simulink model "FCSSystem"  (R2025b)
settings: Solver=VariableStepAuto  StartTime=0.0  StopTime=10.0  RelTol=1e-3
settings Model: DataDictionary=FCSInterfaces.sldd  Creator=sarah  LastModifiedBy=sarah

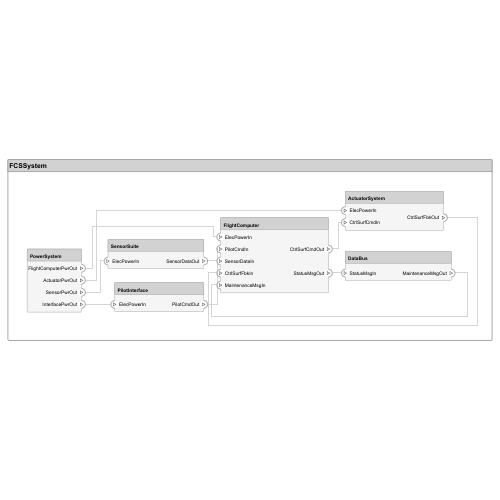
[thumbnail: Simulink's stored preview of the top-level diagram]
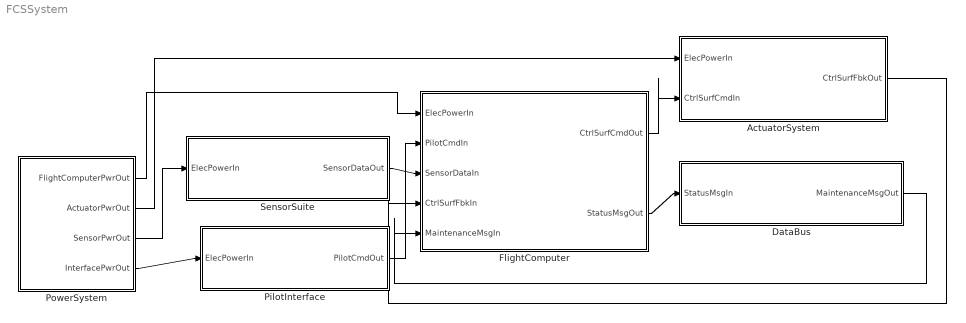
== system FCSSystem ==
  ActuatorSystem : Subsystem
      settings: PortSchema="{\"entries\":[{\"content\":{\"headerSize\":26,\"margin\":15,\"minimumSpacing\":25,\"sides\":[{\"content\":{\"connectorIds\":[\"In1\",\"In2\"]},\"type\":\"ConnectorPlacement.EquallySpacedRectSide\",\"uuid\":\"20d6bed0-d8e5-4088-8794-9345a2942e90\"},{\"content\":{\"connectorIds\":[\"Out1\"],\"side\":\"RIGHT\"},\"type\":\"ConnectorPlacement.EquallySpacedRectSide\",\"uuid\":\"e7adde65-1579-42e2-b600-0f533305a23b\"},{\"content\":{\"side\":\"TOP\"},\"type\":\"ConnectorPlacement.EquallySpacedRectSide\",\"uuid\":\"73636ec6-6908-4b74-b302-6e84b019a70e\"}]},\"type\":\"ConnectorPlacement.EquallySpacedConnector\",\"uuid\":\"cc5d9ea4-0f09-4026-9dcf-92b706ac45bf\"}],\"packageUris\":[\"http://schema.mathworks.com/mf0/Connector/R2020b\"],\"version\":\"1.0\"}"
  DataBus : Subsystem
      settings: PortSchema="{\"entries\":[{\"content\":{\"headerSize\":26,\"margin\":15,\"minimumSpacing\":25,\"sides\":[{\"content\":{\"connectorIds\":[\"In1\"]},\"type\":\"ConnectorPlacement.EquallySpacedRectSide\",\"uuid\":\"20d6bed0-d8e5-4088-8794-9345a2942e90\"},{\"content\":{\"connectorIds\":[\"Out1\"],\"side\":\"RIGHT\"},\"type\":\"ConnectorPlacement.EquallySpacedRectSide\",\"uuid\":\"e7adde65-1579-42e2-b600-0f533305a23b\"},{\"content\":{\"side\":\"TOP\"},\"type\":\"ConnectorPlacement.EquallySpacedRectSide\",\"uuid\":\"73636ec6-6908-4b74-b302-6e84b019a70e\"}]},\"type\":\"ConnectorPlacement.EquallySpacedConnector\",\"uuid\":\"cc5d9ea4-0f09-4026-9dcf-92b706ac45bf\"}],\"packageUris\":[\"http://schema.mathworks.com/mf0/Connector/R2020b\"],\"version\":\"1.0\"}"
  FlightComputer : Subsystem
      settings: PortSchema="{\"entries\":[{\"content\":{\"headerSize\":26,\"margin\":15,\"minimumSpacing\":25,\"sides\":[{\"content\":{\"connectorIds\":[\"In1\",\"In2\",\"In3\",\"In4\",\"In5\"]},\"type\":\"ConnectorPlacement.EquallySpacedRectSide\",\"uuid\":\"20d6bed0-d8e5-4088-8794-9345a2942e90\"},{\"content\":{\"connectorIds\":[\"Out1\",\"Out2\"],\"side\":\"RIGHT\"},\"type\":\"ConnectorPlacement.EquallySpacedRectSide\",\"uuid\":\"e7adde65-1579-42e2-b600-0f533305a23b\"},{\"content\":{\"side\":\"TOP\"},\"type\":\"ConnectorPlacement.EquallySpacedRectSide\",\"uuid\":\"73636ec6-6908-4b74-b302-6e84b019a70e\"}]},\"type\":\"ConnectorPlacement.EquallySpacedConnector\",\"uuid\":\"cc5d9ea4-0f09-4026-9dcf-92b706ac45bf\"}],\"packageUris\":[\"http://schema.mathworks.com/mf0/Connector/R2020b\"],\"version\":\"1.0\"}"
  PilotInterface : Subsystem
      settings: PortSchema="{\"entries\":[{\"content\":{\"headerSize\":26,\"margin\":15,\"minimumSpacing\":25,\"sides\":[{\"content\":{\"connectorIds\":[\"In1\"]},\"type\":\"ConnectorPlacement.EquallySpacedRectSide\",\"uuid\":\"20d6bed0-d8e5-4088-8794-9345a2942e90\"},{\"content\":{\"connectorIds\":[\"Out1\"],\"side\":\"RIGHT\"},\"type\":\"ConnectorPlacement.EquallySpacedRectSide\",\"uuid\":\"e7adde65-1579-42e2-b600-0f533305a23b\"},{\"content\":{\"side\":\"TOP\"},\"type\":\"ConnectorPlacement.EquallySpacedRectSide\",\"uuid\":\"73636ec6-6908-4b74-b302-6e84b019a70e\"}]},\"type\":\"ConnectorPlacement.EquallySpacedConnector\",\"uuid\":\"cc5d9ea4-0f09-4026-9dcf-92b706ac45bf\"}],\"packageUris\":[\"http://schema.mathworks.com/mf0/Connector/R2020b\"],\"version\":\"1.0\"}"
  PowerSystem : Subsystem
      settings: PortSchema="{\"entries\":[{\"content\":{\"headerSize\":26,\"margin\":15,\"minimumSpacing\":25,\"sides\":[{\"content\":{},\"type\":\"ConnectorPlacement.EquallySpacedRectSide\",\"uuid\":\"20d6bed0-d8e5-4088-8794-9345a2942e90\"},{\"content\":{\"connectorIds\":[\"Out1\",\"Out2\",\"Out3\",\"Out4\"],\"side\":\"RIGHT\"},\"type\":\"ConnectorPlacement.EquallySpacedRectSide\",\"uuid\":\"e7adde65-1579-42e2-b600-0f533305a23b\"},{\"content\":{\"side\":\"TOP\"},\"type\":\"ConnectorPlacement.EquallySpacedRectSide\",\"uuid\":\"73636ec6-6908-4b74-b302-6e84b019a70e\"}]},\"type\":\"ConnectorPlacement.EquallySpacedConnector\",\"uuid\":\"cc5d9ea4-0f09-4026-9dcf-92b706ac45bf\"}],\"packageUris\":[\"http://schema.mathworks.com/mf0/Connector/R2020b\"],\"version\":\"1.0\"}"
  SensorSuite : Subsystem
      settings: PortSchema="{\"entries\":[{\"content\":{\"headerSize\":26,\"margin\":15,\"minimumSpacing\":25,\"sides\":[{\"content\":{\"connectorIds\":[\"In1\"]},\"type\":\"ConnectorPlacement.EquallySpacedRectSide\",\"uuid\":\"20d6bed0-d8e5-4088-8794-9345a2942e90\"},{\"content\":{\"connectorIds\":[\"Out1\"],\"side\":\"RIGHT\"},\"type\":\"ConnectorPlacement.EquallySpacedRectSide\",\"uuid\":\"e7adde65-1579-42e2-b600-0f533305a23b\"},{\"content\":{\"side\":\"TOP\"},\"type\":\"ConnectorPlacement.EquallySpacedRectSide\",\"uuid\":\"73636ec6-6908-4b74-b302-6e84b019a70e\"}]},\"type\":\"ConnectorPlacement.EquallySpacedConnector\",\"uuid\":\"cc5d9ea4-0f09-4026-9dcf-92b706ac45bf\"}],\"packageUris\":[\"http://schema.mathworks.com/mf0/Connector/R2020b\"],\"version\":\"1.0\"}"
  wires:
  PowerSystem/4(InterfacePwrOut) -> PilotInterface/1(ElecPowerIn)
  PowerSystem/3(SensorPwrOut) -> SensorSuite/1(ElecPowerIn)
  DataBus/1(MaintenanceMsgOut) -> FlightComputer/5(MaintenanceMsgIn)
  PowerSystem/2(ActuatorPwrOut) -> ActuatorSystem/1(ElecPowerIn)
  PowerSystem/1(FlightComputerPwrOut) -> FlightComputer/1(ElecPowerIn)
  SensorSuite/1(SensorDataOut) -> FlightComputer/3(SensorDataIn)
  PilotInterface/1(PilotCmdOut) -> FlightComputer/2(PilotCmdIn)
  FlightComputer/2(StatusMsgOut) -> DataBus/1(StatusMsgIn)
  FlightComputer/1(CtrlSurfCmdOut) -> ActuatorSystem/2(CtrlSurfCmdIn)
  ActuatorSystem/1(CtrlSurfFbkOut) -> FlightComputer/4(CtrlSurfFbkIn)

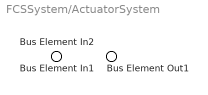
== system FCSSystem/ActuatorSystem ==
  Bus Element In1 : Inport  PortName=ElecPowerIn
  Bus Element In2 : Inport  Port=2  PortName=CtrlSurfCmdIn
  Bus Element Out1 : Outport  PortName=CtrlSurfFbkOut

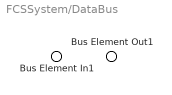
== system FCSSystem/DataBus ==
  Bus Element In1 : Inport  PortName=StatusMsgIn
  Bus Element Out1 : Outport  PortName=MaintenanceMsgOut

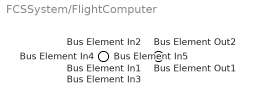
== system FCSSystem/FlightComputer ==
  Bus Element In1 : Inport  PortName=ElecPowerIn
  Bus Element In2 : Inport  Port=2  PortName=PilotCmdIn
  Bus Element In3 : Inport  Port=3  PortName=SensorDataIn
  Bus Element In4 : Inport  Port=4  PortName=CtrlSurfFbkIn
  Bus Element In5 : Inport  Port=5  PortName=MaintenanceMsgIn
  Bus Element Out1 : Outport  PortName=CtrlSurfCmdOut
  Bus Element Out2 : Outport  Port=2  PortName=StatusMsgOut

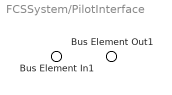
== system FCSSystem/PilotInterface ==
  Bus Element In1 : Inport  PortName=ElecPowerIn
  Bus Element Out1 : Outport  PortName=PilotCmdOut

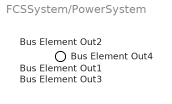
== system FCSSystem/PowerSystem ==
  Bus Element Out1 : Outport  PortName=FlightComputerPwrOut
  Bus Element Out2 : Outport  Port=2  PortName=ActuatorPwrOut
  Bus Element Out3 : Outport  Port=3  PortName=SensorPwrOut
  Bus Element Out4 : Outport  Port=4  PortName=InterfacePwrOut

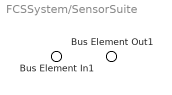
== system FCSSystem/SensorSuite ==
  Bus Element In1 : Inport  PortName=ElecPowerIn
  Bus Element Out1 : Outport  PortName=SensorDataOut
